simulink model "NewtonRaphson_Equation_Solver"  (R2012b)
settings: Solver=FixedStepDiscrete  StartTime=0.0  StopTime=50  FixedStep=1  RelTol=1e-3
libraries: Lib_Solve_SSNRSolverJC_TMATS x1
settings Model: Creator=jwchapm2  LastModifiedBy=jwchapm2
settings OptimizationCC: InlineParams=on  SimCompilerOptimization=On
settings ModelReferenceCC: PropagateVarSize=Only when enabling

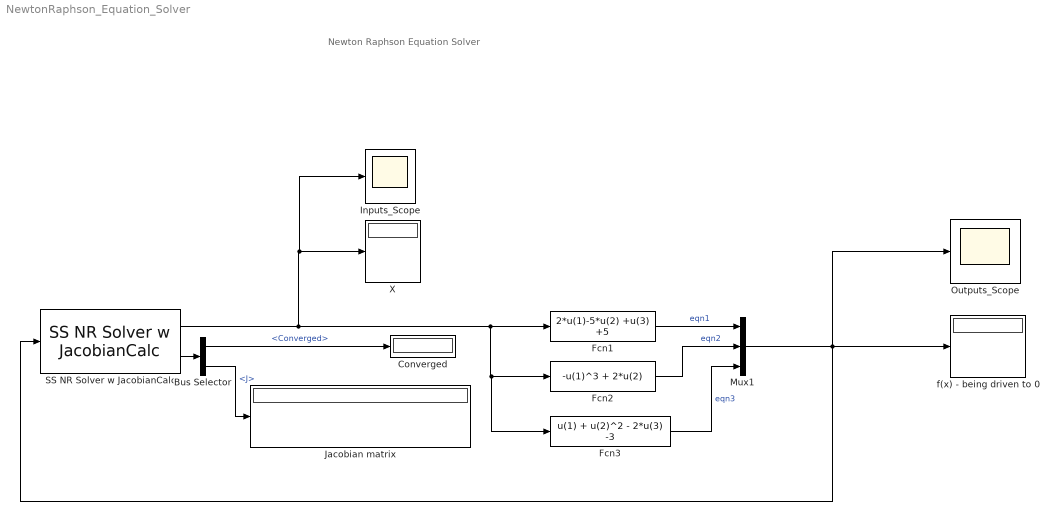
== system NewtonRaphson_Equation_Solver ==
  note: Newton Raphson Equation Solver
  Bus Selector : BusSelector  OutputSignals=Converged,J
  Converged : Display
  Fcn1 : Fcn  Expr=2*u(1)-5*u(2) +u(3) +5
  Fcn2 : Fcn  Expr=-u(1)^3 + 2*u(2)
  Fcn3 : Fcn  Expr=u(1) + u(2)^2 - 2*u(3) -3
  Inputs_Scope : Scope
      settings: ShowLegends=on
  Jacobian matrix : Display
  Mux1 : Mux  Inputs=3
  Outputs_Scope : Scope
      settings: ShowLegends=on  TimeRange=50
  SS NR Solver w JacobianCalc : Lib_Solve_SSNRSolverJC_TMATS/SS NR Solver w JacobianCalc  Priority=1  SJac_Per_M=[0.05; 0.05; 0.05]  SNR_IC_M=[1; 1; 1]  SNR_DX_M=5  SJacobianAttempts_M=20  Cond_Limits_M=0.001
  X : Display
  f(x) - being driven to 0 : Display
  wires:
  Mux1/1 -> Outputs_Scope/1, f(x) - being driven to 0/1, SS NR Solver w JacobianCalc/1
  Fcn1/1 -> Mux1/1  "eqn1"
  Fcn2/1 -> Mux1/2  "eqn2"
  SS NR Solver w JacobianCalc/1 -> Inputs_Scope/1, X/1, Fcn3/1, Fcn2/1, Fcn1/1
  Fcn3/1 -> Mux1/3  "eqn3"
  SS NR Solver w JacobianCalc/2 -> Bus Selector/1
  Bus Selector/1 -> Converged/1  "<Converged>"
  Bus Selector/2 -> Jacobian matrix/1  "<J>"
